simulink model "I_Func_of_F_Two_wires"  (R2021b)
settings: Solver=FixedStepAuto  StartTime=-3000e-6  StopTime=3000e-6  FixedStep=25e-6  RelTol=1e-3
settings Model: Creator=teja  LastModifiedBy=teja

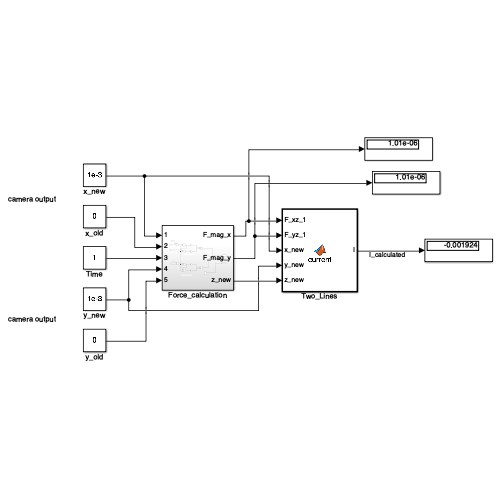
[thumbnail: Simulink's stored preview of the top-level diagram]
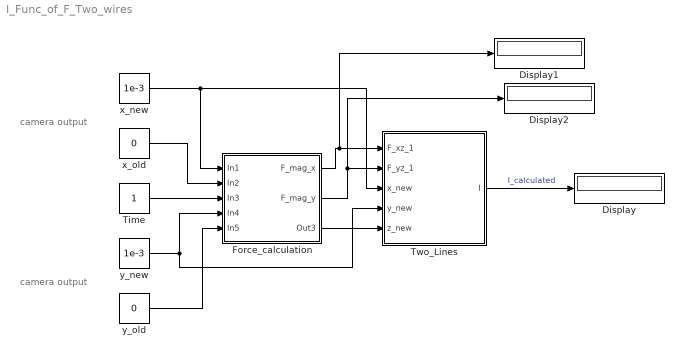
== system I_Func_of_F_Two_wires ==
  note: camera output
  note: camera output
  Display : Display
  Display1 : Display
  Display2 : Display
  Force_calculation : Subsystem
  Time : Constant
  Two_Lines : MATLAB Function  TreatAsAtomicUnit=on
  x_new : Constant  Value=1e-3
  x_old : Constant  Value=0
  y_new : Constant  Value=1e-3
  y_old : Constant  Value=0
  wires:
  x_new/1 -> Force_calculation/1(In1), Two_Lines/3(x_new)
  y_new/1 -> Two_Lines/4(y_new), Force_calculation/4(In4)
  Two_Lines/1(I) -> Display/1  "I_calculated"
  x_old/1 -> Force_calculation/2(In2)
  Time/1 -> Force_calculation/3(In3)
  y_old/1 -> Force_calculation/5(In5)
  Force_calculation/3(Out3) -> Two_Lines/5(z_new)
  Force_calculation/1(F_mag_x) -> Display1/1, Two_Lines/1(F_xz_1)
  Force_calculation/2(F_mag_y) -> Display2/1, Two_Lines/2(F_yz_1)

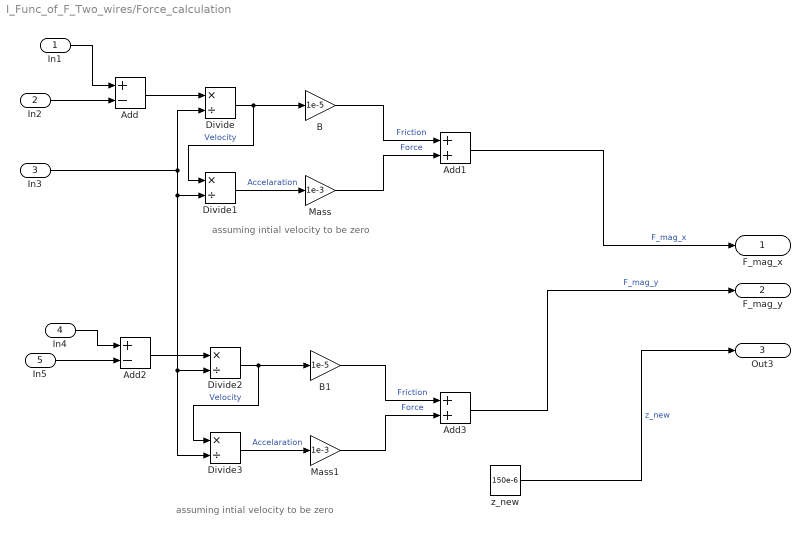
== system I_Func_of_F_Two_wires/Force_calculation ==
  note: assuming intial velocity to be zero
  note: assuming intial velocity to be zero
  In1 : Inport
  In2 : Inport  Port=2
  In3 : Inport  Port=3
  In4 : Inport  Port=4
  In5 : Inport  Port=5
  Add : Sum  Inputs=+-
  Add1 : Sum
  Add2 : Sum  Inputs=+-
  Add3 : Sum
  B : Gain  Gain=1e-5
  B1 : Gain  Gain=1e-5
  Divide{,1..3} (4 alike) : Product  Inputs=*/
  Mass : Gain  Gain=1e-3
  Mass1 : Gain  Gain=1e-3
  z_new : Constant  Value=150e-6
  F_mag_x : Outport
  F_mag_y : Outport  Port=2
  Out3 : Outport  Port=3
  wires:
  In4/1 -> Add2/1
  z_new/1 -> Out3/1  "z_new"
  Add3/1 -> F_mag_y/1  "F_mag_y"
  Add1/1 -> F_mag_x/1  "F_mag_x"
  In5/1 -> Add2/2
  Mass/1 -> Add1/2  "Force"
  Add2/1 -> Divide2/1
  B1/1 -> Add3/1  "Friction"
  Mass1/1 -> Add3/2  "Force"
  B/1 -> Add1/1  "Friction"
  In1/1 -> Add/1
  Divide/1 -> Divide1/1, B/1  "Velocity"
  Add/1 -> Divide/1
  Divide2/1 -> B1/1, Divide3/1  "Velocity"
  Divide3/1 -> Mass1/1  "Accelaration"
  Divide1/1 -> Mass/1  "Accelaration"
  In3/1 -> Divide3/2, Divide2/2, Divide1/2, Divide/2
  In2/1 -> Add/2

== matlab function I_Func_of_F_Two_wires/Two_Lines ==
  data: I output; F_xz_1 input; F_yz_1 input; x_new input; y_new input; z_new input
function  I = current( F_xz_1, F_yz_1, x_new, y_new, z_new)

g = 200e-6;     %Coil spacing
m0 = 4*pi*1e-7;
radius = 3e-3;%m
height = 1e-3;%m
Magentization = 1.45; %T
vol_cy = pi*radius^2*height; % If Object is Cylinder, vol in m^3
% vol_sp = (4/3)*(pi * radius^3); % If Object is Sphere, vol in m^3

k = 0.4e-3; %additional length added to wires, to get concentric coil
%--------%--------%--------%--------%--------%--------%--------%----------
% Line along y - axis
%-%--------%--------%--------%--------%--------%--------%--------%--------
y1_1 = -0.6e-3;
y2_1 = 0.6e-3;
a_xp_1 = g;  
a_xn_1 = -g;

k_yp_1 = 1/(4*pi*((a_xp_1-x_new)^2+z_new^2));
k_1yp_1 = (y2_1-y_new)/((y2_1-y_new)^2+(a_xp_1-x_new)^2+z_new^2)^0.5;
k_2yp_1 = (y1_1-y_new)/((y1_1-y_new)^2+(a_xp_1-x_new)^2+z_new^2)^0.5;

k_1yp_3 = (y2_1-y_new)/((y2_1-y_new)^2+(a_xp_1-x_new)^2+z_new^2)^1.5;
k_2yp_3 = (y1_1-y_new)/((y1_1-y_new)^2+(a_xp_1-x_new)^2+z_new^2)^1.5;

k_yn_1 = 1/(4*pi*((a_xn_1-x_new)^2+z_new^2));
k_1yn_1 = (y2_1-y_new)/((y2_1-y_new)^2+(a_xn_1-x_new)^2+z_new^2)^0.5;
k_2yn_1 = (y1_1-y_new)/((y1_1-y_new)^2+(a_xn_1-x_new)^2+z_new^2)^0.5;

k_1yn_3 = (y2_1-y_new)/((y2_1-y_new)^2+(a_xn_1-x_new)^2+z_new^2)^1.5;
k_2yn_3 = (y1_1-y_new)/((y1_1-y_new)^2+(a_xn_1-x_new)^2+z_new^2)^1.5;

hyp_x_1 = -(z_new*k_yp_1*(a_xp_1-x_new)) *m0;
hyp_x1_1 = (k_yp_1*(k_1yp_1 - k_2yp_1))*2*4*pi;
hyp_x2_1 = k_1yp_3 - k_2yp_3;
dBxp_1_dx = hyp_x_1*(hyp_x1_1 + hyp_x2_1);

hyp_z_1 = (k_yp_1) *m0;
hyp_z1_1 = (k_1yp_1 - k_2yp_1)*(-1);
hyp_z2_1 = (k_yp_1*(k_1yp_1 - k_2yp_1)*(z_new^2))*4*pi*2;
hyp_z3_1 = (k_1yp_3 - k_2yp_3)*(z_new^2);
dBxp_1_dz = hyp_z_1*(hyp_z1_1 + hyp_z2_1 + hyp_z3_1);

hyn_x_1 = -(z_new*k_yn_1*(a_xn_1-x_new)) *m0*(-1);
hyn_x1_1 = (k_yn_1*(k_1yn_1 - k_2yn_1))*2*4*pi;
hyn_x2_1 = k_1yn_3 - k_2yn_3;
dBxn_1_dx = hyn_x_1*(hyn_x1_1 + hyn_x2_1);

hyn_z_1 = (k_yn_1)* m0*(-1);
hyn_z1_1 = (k_1yn_1 - k_2yn_1)*(-1);
hyn_z2_1 = (k_yn_1*(k_1yn_1 - k_2yn_1)*(z_new^2))*4*pi*2;
hyn_z3_1 = (k_1yn_3 - k_2yn_3)*(z_new^2);
dBxn_1_dz = hyn_z_1*(hyn_z1_1 + hyn_z2_1 + hyn_z3_1);

%--------%--------%--------%--------%--------%--------%--------%----------
% Line along x - axis
%-%--------%--------%--------%--------%a--------%--------%--------%--------
x1_1 = -0.6e-3;
x2_1 = 0.6e-3;
a_yp_1 = g;          %Distance of coil from (0,0)
a_yn_1 = -g;

k_xp_1 = 1/(4*pi*((a_yp_1-y_new)^2+z_new^2));
k_1xp_1 = (x2_1-x_new)/((x2_1-x_new)^2+(a_yp_1-y_new)^2+z_new^2)^0.5;
k_2xp_1 = (x1_1-x_new)/((x1_1-x_new)^2+(a_yp_1-y_new)^2+z_new^2)^0.5;

k_xn_1 = 1/(4*pi*((a_yn_1-y_new)^2+z_new^2));
k_1xn_1 = (x2_1-x_new)/((x2_1-x_new)^2+(a_yn_1-y_new)^2+z_new^2)^0.5;
k_2xn_1 = (x1_1-x_new)/((x1_1-x_new)^2+(a_yn_1-y_new)^2+z_new^2)^0.5;

k_1xp_3 = (x2_1-x_new)/((x2_1-x_new)^2+(a_yp_1-y_new)^2+z_new^2)^1.5;
k_2xp_3 = (x1_1-x_new)/((x1_1-x_new)^2+(a_yp_1-y_new)^2+z_new^2)^1.5;

k_1xn_3 = (x2_1-x_new)/((x2_1-x_new)^2+(a_yn_1-y_new)^2+z_new^2)^1.5;
k_2xn_3 = (x1_1-x_new)/((x1_1-x_new)^2+(a_yn_1-y_new)^2+z_new^2)^1.5;

hxp_x_1 = -(z_new*k_xp_1*(a_yp_1-y_new))*m0;
hxp_x1_1 = (k_xp_1*(k_1xp_1 - k_2xp_1))*2*4*pi;
hxp_x2_1 = k_1xp_3 - k_2xp_3;
dByp_1_dy = hxp_x_1*(hxp_x1_1 + hxp_x2_1);

hxp_z_1 = (k_xp_1)*m0;
hxp_z1_1 = (k_1xp_1 - k_2xp_1)*(-1);
hxp_z2_1 = (k_xp_1*(k_1xp_1 - k_2xp_1)*(z_new^2))*4*pi*2;
hxp_z3_1 = (k_1xp_3 - k_2xp_3)*(z_new^2);
dByp_1_dz = hxp_z_1*(hxp_z1_1 + hxp_z2_1 + hxp_z3_1);

hxn_x_1 = -(z_new*k_xn_1*(a_yn_1-y_new))*m0*(-1);
hxn_x1_1 = (k_xn_1*(k_1xn_1 - k_2xn_1))*2*4*pi;
hxn_x2_1 = k_1xn_3 - k_2xn_3;
dByn_1_dy = hxn_x_1*(hxn_x1_1 + hxn_x2_1);

hxn_z_1 = (k_xn_1)*m0*(-1);
hxn_z1_1 = (k_1xn_1 - k_2xn_1)*(-1);
hxn_z2_1 = (k_xn_1*(k_1xn_1 - k_2xn_1)*(z_new^2))*4*pi*2;
hxn_z3_1 = (k_1xn_3 - k_2xn_3)*(z_new^2);
dByn_1_dz = hxn_z_1*(hxn_z1_1 + hxn_z2_1 + hxn_z3_1);

I = (F_xz_1/ (dBxp_1_dz + dBxn_1_dz)+  F_yz_1 / (dByp_1_dz + dByn_1_dz))* m0/ (vol_cy * Magentization);
end
